simulink model "Task26"  (R2025a)
settings: Solver=VariableStepAuto  StartTime=0.0  StopTime=10.0  RelTol=1e-3
settings Model: Creator=LOQ  LastModifiedBy=LOQ

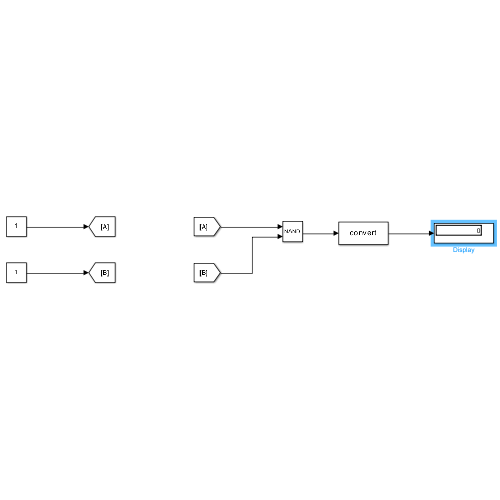
[thumbnail: Simulink's stored preview of the top-level diagram]
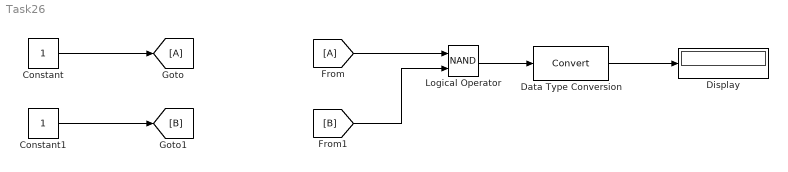
== system Task26 ==
  Constant : Constant  OutDataTypeStr=boolean
  Constant1 : Constant  OutDataTypeStr=boolean
  Data Type Conversion : DataTypeConversion  SaturateOnIntegerOverflow=off  RndMeth=Floor
  Display : Display
  From : From
  Goto : Goto
  Logical Operator : Logic  Operator=NAND  AllPortsSameDT=off  OutDataTypeStr=boolean
  wires:
  Constant1/1 -> [B]
  Constant/1 -> Goto/1
  Data Type Conversion/1 -> Display/1
  From/1 -> Logical Operator/1
  [B] -> Logical Operator/2
  Logical Operator/1 -> Data Type Conversion/1
